simulink model "sistemadiscretowindup"  (Simulink 4.00)
settings: Solver=ode45  StartTime=0.0  StopTime=2  MaxStep=0.0001  RelTol=1e-3
settings Model: LastModifiedBy=Gui  RTWOptions="-aEnforceIntegerDowncast=1 -aExtMode=0 -aFoldNonRolledExpr=1 -aForceParamTrailComments=0 -aGenerateComments=1 -aIgnoreCustomStorageClasses=1 -aIncHierarchyInIds=0 -aInlineInvariantSignals=0 -aLocalBlockOutputs=1 -aLogVarNameModifier=\"rt_\" -aRTWVerbose=1 -aRollThreshold=5 -aShowEliminatedStatements=1"

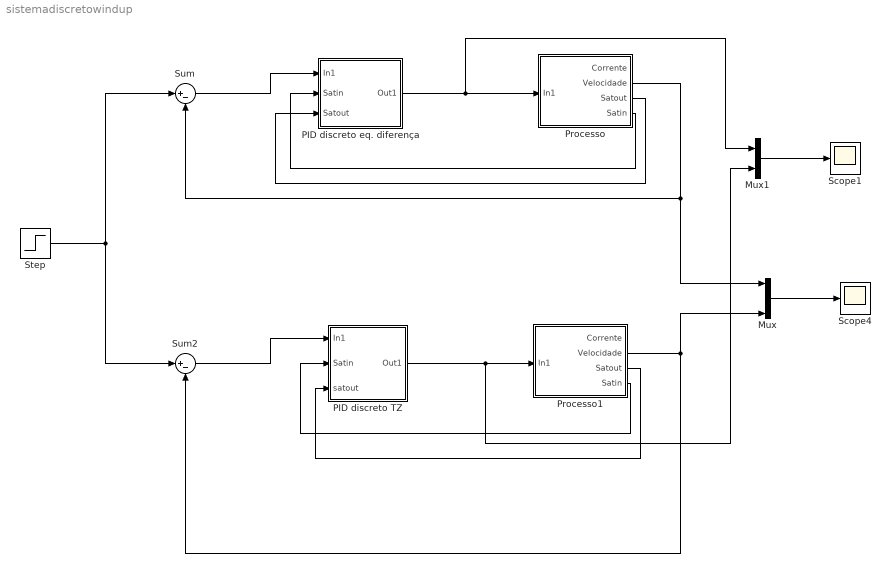
== system sistemadiscretowindup ==
  Mux : Mux  Inputs=3
  Mux1 : Mux  Inputs=2
  PID discreto TZ : Subsystem
      settings: RTWFcnNameOpts=Auto  RTWFileNameOpts=Auto
  "PID discreto eq. diferença " : Subsystem
      settings: RTWFcnNameOpts=Auto  RTWFileNameOpts=Auto
  Processo : Subsystem
      settings: RTWFcnNameOpts=Auto  RTWFileNameOpts=Auto
  Processo1 : Subsystem
      settings: RTWFcnNameOpts=Auto  RTWFileNameOpts=Auto
  Scope1 : Scope
      settings: TimeRange=0.05  YMin=0.5  YMax=7  SaveToWorkspace=off  SaveName=ScopeData  MaxDataPoints=5000
  Scope4 : Scope
      settings: TimeRange=2  YMin=-0.5  YMax=2.5  SaveToWorkspace=off  SaveName=ScopeData2  MaxDataPoints=5000
  Step : Step  Time=0.12  Before=0  After=1  SampleTime=0
  Sum : Sum  Inputs=|+-  SaturateOnIntegerOverflow=on
  Sum2 : Sum  Inputs=|+-  SaturateOnIntegerOverflow=on
  wires:
  Sum/1 -> "PID discreto eq. diferença "/1(In1)
  Mux/1 -> Scope4/1
  Sum2/1 -> PID discreto TZ/1(In1)
  "PID discreto eq. diferença "/1(Out1) -> Processo/1(In1), Mux1/1
  PID discreto TZ/1(Out1) -> Processo1/1(In1), Mux1/2
  Processo/2(Velocidade) -> Sum/2, Mux/1
  Processo1/2(Velocidade) -> Sum2/2, Mux/3
  Step/1 -> Sum/1, Sum2/1
  Mux1/1 -> Scope1/1
  Processo/4(Satin) -> "PID discreto eq. diferença "/2(Satin)
  Processo/3(Satout) -> "PID discreto eq. diferença "/3(Satout)
  Processo1/4(Satin) -> PID discreto TZ/2(Satin)
  Processo1/3(Satout) -> PID discreto TZ/3(satout)

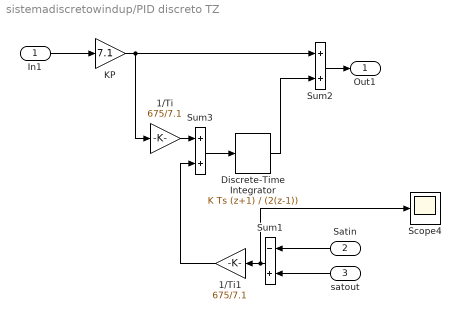
== system sistemadiscretowindup/PID discreto TZ ==
  In1 : Inport  Port=1  LatchInput=off  SampleTime=0.005
  Satin : Inport  Orientation=left  Port=2  LatchInput=off  SampleTime=0.005
  satout : Inport  Orientation=left  Port=3  LatchInput=off  SampleTime=0.005
  1/Ti : Gain  Gain=675/7.1  Multiplication=Element-wise(K.*u)  SaturateOnIntegerOverflow=on
  1/Ti1 : Gain  Orientation=left  Gain=675/7.1  Multiplication=Element-wise(K.*u)  SaturateOnIntegerOverflow=on
  Discrete-Time Integrator : DiscreteIntegrator  IntegratorMethod=Trapezoidal  ExternalReset=none  InitialConditionSource=internal  InitialCondition=0  LimitOutput=off  UpperSaturationLimit=inf  LowerSaturationLimit=-inf  ShowSaturationPort=off  ShowStatePort=off  SampleTime=0.005
      settings: RTWStateStorageClass=Auto
  KP : Gain  Gain=7.1  Multiplication=Element-wise(K.*u)  SaturateOnIntegerOverflow=on
  Scope4 : Scope
      settings: TimeRange=0.05  YMin=0.5  YMax=7  SaveToWorkspace=off  SaveName=ScopeData3  MaxDataPoints=5000
  Sum1 : Sum  Orientation=left  Inputs=-+  SaturateOnIntegerOverflow=on
  Sum2 : Sum  Inputs=++  SaturateOnIntegerOverflow=on
  Sum3 : Sum  Inputs=++  SaturateOnIntegerOverflow=on
  Out1 : Outport  Port=1
  wires:
  Sum2/1 -> Out1/1
  KP/1 -> Sum2/1, 1/Ti/1
  In1/1 -> KP/1
  Discrete-Time Integrator/1 -> Sum2/2
  Satin/1 -> Sum1/1
  satout/1 -> Sum1/2
  1/Ti/1 -> Sum3/1
  Sum3/1 -> Discrete-Time Integrator/1
  Sum1/1 -> 1/Ti1/1, Scope4/1
  1/Ti1/1 -> Sum3/2

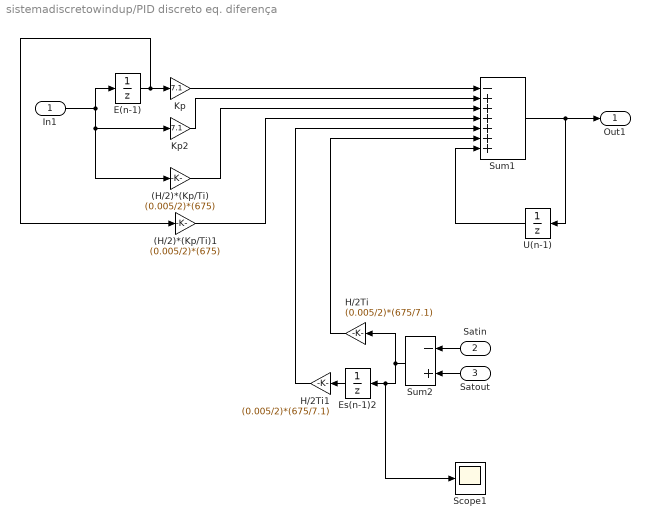
== system sistemadiscretowindup/PID discreto eq. diferença  ==
  In1 : Inport  Port=1  LatchInput=off  SampleTime=0.005
  Satin : Inport  Orientation=left  Port=2  LatchInput=off  SampleTime=0.005
  Satout : Inport  Orientation=left  Port=3  LatchInput=off  SampleTime=0.005
  (H/2)*(Kp/Ti) : Gain  Gain=(0.005/2)*(675)  Multiplication=Element-wise(K.*u)  SaturateOnIntegerOverflow=on
  (H/2)*(Kp/Ti)1 : Gain  Gain=(0.005/2)*(675)  Multiplication=Element-wise(K.*u)  SaturateOnIntegerOverflow=on
  E(n-1) : UnitDelay  X0=0  SampleTime=0.005
      settings: RTWStateStorageClass=Auto
  Es(n-1)2 : UnitDelay  Orientation=left  X0=0  SampleTime=0.005
      settings: RTWStateStorageClass=Auto
  H/2Ti : Gain  Orientation=left  Gain=(0.005/2)*(675/7.1)  Multiplication=Element-wise(K.*u)  SaturateOnIntegerOverflow=on
  H/2Ti1 : Gain  Orientation=left  Gain=(0.005/2)*(675/7.1)  Multiplication=Element-wise(K.*u)  SaturateOnIntegerOverflow=on
  Kp : Gain  Gain=7.1  Multiplication=Element-wise(K.*u)  SaturateOnIntegerOverflow=on
  Kp2 : Gain  Gain=7.1  Multiplication=Element-wise(K.*u)  SaturateOnIntegerOverflow=on
  Scope1 : Scope
      settings: TimeRange=0.05  YMin=0.5  YMax=7  SaveToWorkspace=off  MaxDataPoints=5000
  Sum1 : Sum  Inputs=-++++++  SaturateOnIntegerOverflow=on
  Sum2 : Sum  Orientation=left  Inputs=-+  SaturateOnIntegerOverflow=on
  U(n-1) : UnitDelay  Orientation=left  X0=0  SampleTime=0.005
      settings: RTWStateStorageClass=Auto
  Out1 : Outport  Port=1
  wires:
  Sum1/1 -> U(n-1)/1, Out1/1
  Satin/1 -> Sum2/1
  Satout/1 -> Sum2/2
  In1/1 -> Kp2/1, (H/2)*(Kp/Ti)/1, E(n-1)/1
  E(n-1)/1 -> Kp/1, (H/2)*(Kp/Ti)1/1
  U(n-1)/1 -> Sum1/7
  Sum2/1 -> H/2Ti/1, Es(n-1)2/1, Scope1/1
  H/2Ti/1 -> Sum1/6
  Es(n-1)2/1 -> H/2Ti1/1
  H/2Ti1/1 -> Sum1/5
  Kp2/1 -> Sum1/2
  (H/2)*(Kp/Ti)/1 -> Sum1/3
  (H/2)*(Kp/Ti)1/1 -> Sum1/4
  Kp/1 -> Sum1/1

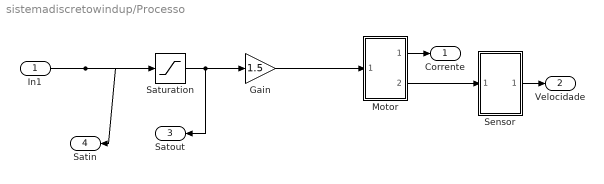
== system sistemadiscretowindup/Processo ==
  In1 : Inport  Port=1  LatchInput=off  SampleTime=0
  Gain : Gain  Gain=1.5  Multiplication=Element-wise(K.*u)  SaturateOnIntegerOverflow=on
  Motor : Subsystem
      settings: RTWFcnNameOpts=Auto  RTWFileNameOpts=Auto
  Saturation : Saturate  UpperLimit=9  LowerLimit=-9  LinearizeAsGain=on
  Sensor : Subsystem
      settings: RTWFcnNameOpts=Auto  RTWFileNameOpts=Auto
  Corrente : Outport  Port=1
  Velocidade : Outport  Port=2
  Satout : Outport  Orientation=left  Port=3
  Satin : Outport  Orientation=left  Port=4
  wires:
  Motor/2(Out2) -> Sensor/1(In1)
  Motor/1(Out1) -> Corrente/1
  Sensor/1(Out1) -> Velocidade/1
  Gain/1 -> Motor/1(In1)
  In1/1 -> Saturation/1, Satin/1
  Saturation/1 -> Gain/1, Satout/1

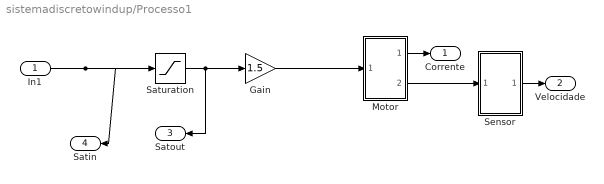
== system sistemadiscretowindup/Processo1 ==
  In1 : Inport  Port=1  LatchInput=off  SampleTime=0
  Gain : Gain  Gain=1.5  Multiplication=Element-wise(K.*u)  SaturateOnIntegerOverflow=on
  Motor : Subsystem
      settings: RTWFcnNameOpts=Auto  RTWFileNameOpts=Auto
  Saturation : Saturate  UpperLimit=9  LowerLimit=-9  LinearizeAsGain=on
  Sensor : Subsystem
      settings: RTWFcnNameOpts=Auto  RTWFileNameOpts=Auto
  Corrente : Outport  Port=1
  Velocidade : Outport  Port=2
  Satout : Outport  Orientation=left  Port=3
  Satin : Outport  Orientation=left  Port=4
  wires:
  Motor/2(Out2) -> Sensor/1(In1)
  Motor/1(Out1) -> Corrente/1
  Sensor/1(Out1) -> Velocidade/1
  Gain/1 -> Motor/1(In1)
  In1/1 -> Saturation/1, Satin/1
  Saturation/1 -> Gain/1, Satout/1

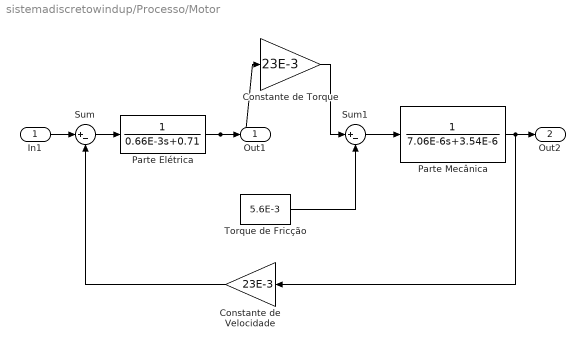
== system sistemadiscretowindup/Processo/Motor ==
  In1 : Inport  Port=1  LatchInput=off  SampleTime=0
  Constante de Torque : Gain  Gain=23E-3  Multiplication=Element-wise(K.*u)  SaturateOnIntegerOverflow=on
  Constante de Velocidade : Gain  Orientation=left  Gain=23E-3  Multiplication=Element-wise(K.*u)  SaturateOnIntegerOverflow=on
  Parte Elétrica : TransferFcn  Numerator=[1]  Denominator=[0.66E-3 0.71]  AbsoluteTolerance=auto  Realization=auto
  Parte Mecânica : TransferFcn  Numerator=[1]  Denominator=[7.06E-6 3.54E-6]  AbsoluteTolerance=auto  Realization=auto
  Sum : Sum  Inputs=|+-  SaturateOnIntegerOverflow=on
  Sum1 : Sum  Inputs=|+-  SaturateOnIntegerOverflow=on
  Torque de Fricção : Constant  Value=5.6E-3
  Out1 : Outport  Port=1
  Out2 : Outport  Port=2
  wires:
  Sum/1 -> Parte Elétrica/1
  Parte Elétrica/1 -> Constante de Torque/1, Out1/1
  Parte Mecânica/1 -> Constante de Velocidade/1, Out2/1
  Constante de Velocidade/1 -> Sum/2
  Constante de Torque/1 -> Sum1/1
  Sum1/1 -> Parte Mecânica/1
  Torque de Fricção/1 -> Sum1/2
  In1/1 -> Sum/1

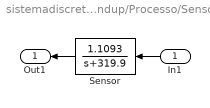
== system sistemadiscretowindup/Processo/Sensor ==
  In1 : Inport  Orientation=left  Port=1  LatchInput=off
  "Sensor " : TransferFcn  Orientation=left  Numerator=[1.1093]  Denominator=[1 319.9]  AbsoluteTolerance=auto  Realization=auto
  Out1 : Outport  Orientation=left  Port=1
  wires:
  "Sensor "/1 -> Out1/1
  In1/1 -> "Sensor "/1

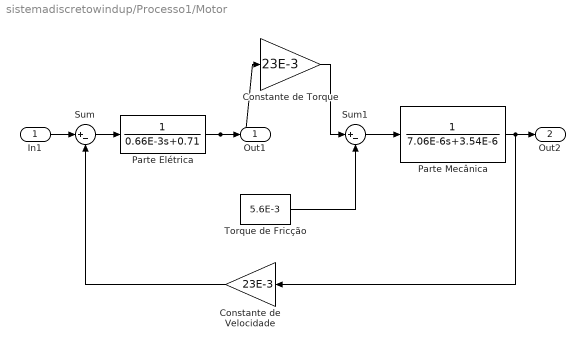
== system sistemadiscretowindup/Processo1/Motor ==
  In1 : Inport  Port=1  LatchInput=off  SampleTime=0
  Constante de Torque : Gain  Gain=23E-3  Multiplication=Element-wise(K.*u)  SaturateOnIntegerOverflow=on
  Constante de Velocidade : Gain  Orientation=left  Gain=23E-3  Multiplication=Element-wise(K.*u)  SaturateOnIntegerOverflow=on
  Parte Elétrica : TransferFcn  Numerator=[1]  Denominator=[0.66E-3 0.71]  AbsoluteTolerance=auto  Realization=auto
  Parte Mecânica : TransferFcn  Numerator=[1]  Denominator=[7.06E-6 3.54E-6]  AbsoluteTolerance=auto  Realization=auto
  Sum : Sum  Inputs=|+-  SaturateOnIntegerOverflow=on
  Sum1 : Sum  Inputs=|+-  SaturateOnIntegerOverflow=on
  Torque de Fricção : Constant  Value=5.6E-3
  Out1 : Outport  Port=1
  Out2 : Outport  Port=2
  wires:
  Sum/1 -> Parte Elétrica/1
  Parte Elétrica/1 -> Constante de Torque/1, Out1/1
  Parte Mecânica/1 -> Constante de Velocidade/1, Out2/1
  Constante de Velocidade/1 -> Sum/2
  Constante de Torque/1 -> Sum1/1
  Sum1/1 -> Parte Mecânica/1
  Torque de Fricção/1 -> Sum1/2
  In1/1 -> Sum/1

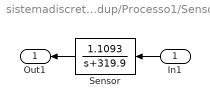
== system sistemadiscretowindup/Processo1/Sensor ==
  In1 : Inport  Orientation=left  Port=1  LatchInput=off
  "Sensor " : TransferFcn  Orientation=left  Numerator=[1.1093]  Denominator=[1 319.9]  AbsoluteTolerance=auto  Realization=auto
  Out1 : Outport  Orientation=left  Port=1
  wires:
  "Sensor "/1 -> Out1/1
  In1/1 -> "Sensor "/1
